simulink model "lee_att_controller"  (R2023a)
settings: Solver=VariableStepAuto  StartTime=0.0  StopTime=10.0  RelTol=1e-3
undefined symbols (not defined in the file): K_o, K_r
settings Model: Creator=jonas  LastModifiedBy=jonas

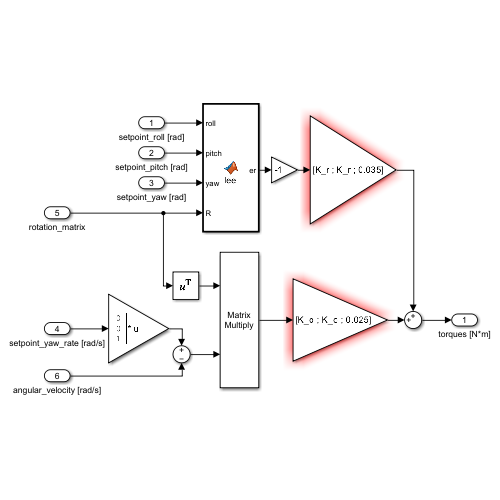
[thumbnail: Simulink's stored preview of the top-level diagram]
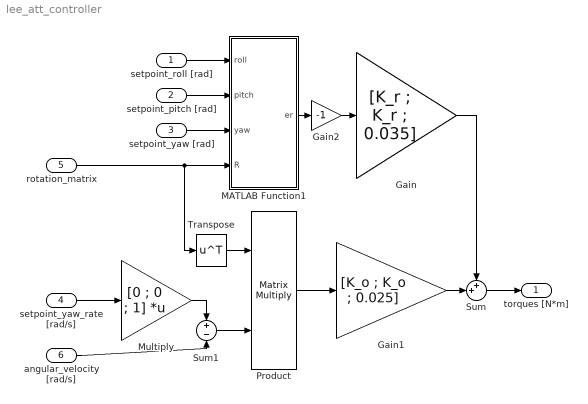
== system lee_att_controller ==
  setpoint_roll [rad] : Inport
  setpoint_pitch [rad] : Inport  Port=2
  setpoint_yaw [rad] : Inport  Port=3
  setpoint_yaw_rate [rad/s] : Inport  Port=4
  rotation_matrix : Inport  Port=5
  angular_velocity [rad/s] : Inport  Port=6
  Gain : Gain  Gain=[K_r ; K_r ; 0.035]
  Gain1 : Gain  Gain=[K_o ; K_o ; 0.025]
  Gain2 : Gain  Gain=-1
  MATLAB Function1 : MATLAB Function  TreatAsAtomicUnit=on
  Multiply : Gain  Gain=[0 ; 0 ; 1]  Multiplication=Matrix(K*u)
  Product : Product  Multiplication=Matrix(*)
  Sum : Sum  Inputs=++|
  Sum1 : Sum  Inputs=+|-
  Transpose : Math  Operator=transpose
  torques [N*m] : Outport
  wires:
  Sum/1 -> torques [N*m]/1
  Gain1/1 -> Sum/2
  Product/1 -> Gain1/1
  Multiply/1 -> Sum1/1
  rotation_matrix/1 -> Transpose/1, MATLAB Function1/4(R)
  setpoint_yaw_rate [rad/s]/1 -> Multiply/1
  angular_velocity [rad/s]/1 -> Sum1/2
  setpoint_roll [rad]/1 -> MATLAB Function1/1(roll)
  setpoint_pitch [rad]/1 -> MATLAB Function1/2(pitch)
  Sum1/1 -> Product/2
  Transpose/1 -> Product/1
  Gain/1 -> Sum/1
  setpoint_yaw [rad]/1 -> MATLAB Function1/3(yaw)
  MATLAB Function1/1(er) -> Gain2/1
  Gain2/1 -> Gain/1

== matlab function lee_att_controller/MATLAB Function1 ==
  data: roll input size=1; pitch input size=1; yaw input size=1; er output size=[3 1]; R input size=[3 3]
function er = lee(roll, pitch, yaw, R)

Rd = eul2rotm([yaw pitch roll], 'ZYX');

P = 1/2 * (Rd.' * R - R.' * Rd) ;

er = [P(3,2) ; P(1,3) ; P(2,1)] ;
